simulink model "add_delay"  (R2020a)
settings: Solver=VariableStepAuto  StartTime=0.0  StopTime=10.0  RelTol=1e-3
libraries: hdlsllib x2
settings Model: Creator=sunip  LastModifiedBy=sunip
settings OptimizationCC: BlockReduction=off  ConditionallyExecuteInputs=off  DefaultParameterBehavior=Inlined  SimCompilerOptimization=on
settings DebuggingCC: AlgebraicLoopMsg=none
settings HardwareCC: ProdBitPerPointer=32  ProdBitPerSizeT=32  ProdBitPerPtrDiffT=32  ProdLargestAtomicFloat=None  ProdIntDivRoundTo=Undefined  ProdEndianess=Unspecified  ProdWordSize=32  ProdHWDeviceType=ASIC/FPGA->ASIC/FPGA  TargetBitPerLong=64  TargetBitPerPointer=64  TargetBitPerSizeT=64  TargetBitPerPtrDiffT=64  TargetLongLongMode=on  TargetIntDivRoundTo=Zero  TargetEndianess=LittleEndian  TargetWordSize=64  TargetHWDeviceType=Custom Processor->MATLAB Host Computer  ProdEqTarget=off

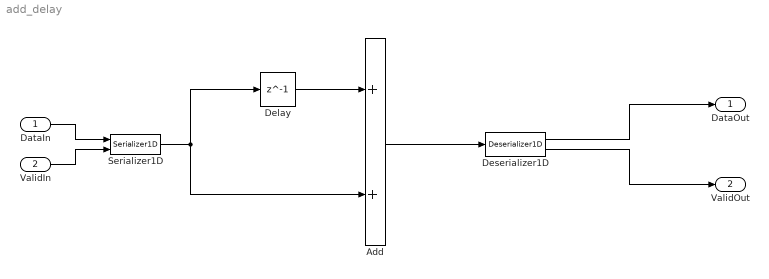
== system add_delay ==
  DataIn : Inport  OutDataTypeStr=uint8  SampleTime=0.001
  ValidIn : Inport  Port=2  OutDataTypeStr=boolean  SampleTime=0.001
  Add : Sum  AccumDataTypeStr=uint8  OutDataTypeStr=uint8
  Delay : Delay  DelayLength=1
  Deserializer1D : hdlsllib/HDL Operations/Deserializer1D  Ratio=1  IdleCycles=0  InitialCondition=0  startIn=off  validIn=off  validOut=on  inputDataDimensions=-1  inputSampleTime=-1  inputSignalType=auto
      settings: SourceProductBaseCode=SL
  Serializer1D : hdlsllib/HDL Operations/Serializer1D  Ratio=1  IdleCycles=0  validIn=on  startOut=off  validOut=off  inputDataDimensions=-1  inputSampleTime=-1  inputSignalType=auto
      settings: SourceProductBaseCode=SL
  DataOut : Outport  OutDataTypeStr=uint8
  ValidOut : Outport  Port=2  OutDataTypeStr=boolean
  wires:
  Add/1 -> Deserializer1D/1
  DataIn/1 -> Serializer1D/1
  Serializer1D/1 -> Delay/1, Add/2
  Deserializer1D/2 -> ValidOut/1
  Deserializer1D/1 -> DataOut/1
  Delay/1 -> Add/1
  ValidIn/1 -> Serializer1D/2
